simulink model "VVA_pressure_dynamic_basefreq"  (R2023b)
settings: Solver=FixedStepAuto  StartTime=0.0  StopTime=0.6  MaxStep=1e-3  RelTol=1e-3
values from neighbouring files (symbols this model uses):
  x = [2*10^5	3*10^5	4*10^5	5*10^5	6*10^5	7*10^5	8*10^5]    [Q.m]    (also in new_run_compare_export_jieyue.m = ts.Data(:); new_run_compare_sin_export.m = ts.Data(:); objfun_ga.m = double(x(:)); run_compare_jieyue.m = ts.Data(:))
  y = [0 ... (first row only)    [Q.m]    (also in new_run_compare_export_jieyue.m = interp1(t0u, x0u, t(:), method, 'extrap'); new_run_compare_sin_export.m = interp1(t0u, x0u, t(:), method, 'extrap'); objfun_ga.m = y(ia); run_compare_jieyue.m = interp1(t0u, x0u, t(:), method, 'extrap'))
  z = [0.893557423	1.334431826	1.76701406	2.210901891	2.65062	3.098039216	3.535707573 ... (first row only)    [Q.m]
undefined symbols (not defined in the file or in its folder): freq_mode
libraries: fuzblock x2, simulink x2
settings Model: Creator=Administrator  LastModifiedBy=47371
settings SolverCC: MaxConsecutiveMinStep=2  ZeroCrossAlgorithm=Adaptive  AlgebraicLoopSolver=TrustRegion
settings DebuggingCC: MaskedZcDiagnostic=none  IgnoredZcDiagnostic=none  ArithmeticOperatorsInVariantConditions=warning
settings SFSimCC: CustomCodeUndefinedFunction=UseInterfaceOnly

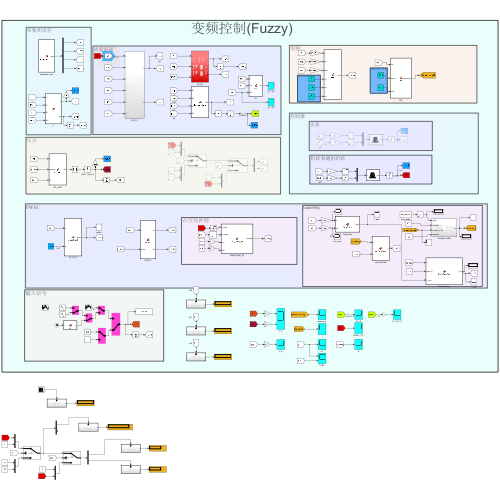
[thumbnail: Simulink's stored preview of the top-level diagram]
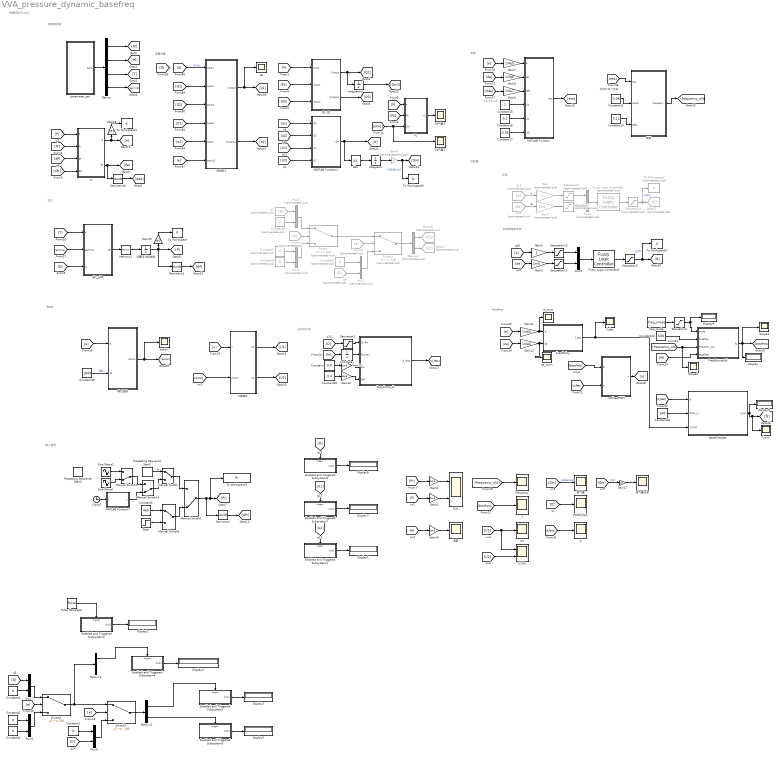
== system VVA_pressure_dynamic_basefreq ==
  note: 输入信号
  note: 占空比补偿
  note: 正弦
  note: 阶跃和随机阶跃
  note: 变频控制(Fuzzy)
  note: 变频
  note: basefrep
  note: 控制器
  note: 压力
  note: 参数和误差
  note: 质量流量
  note: PWM
  note: 变频的两个参数
  note: w1,w2,w3
  2阀模式 : MATLAB Function  TreatAsAtomicUnit=on  SystemSampleTime=0.001
  Abs : Abs  SaturateOnIntegerOverflow=off
  BaseFreqOpt : MATLAB Function  TreatAsAtomicUnit=on
  Clock5 : Clock
  Constant : Constant  Value=0.8
  Constant1 : Constant  Value=4e5
  Constant10 : Constant  Value=1000
  Constant11 : Constant  Value=0.06
  Constant12 : Constant  Value=500
  Constant13 : Constant  Value=500
  Constant14 : Constant  Value=0.12
  Constant15 : Constant
  Constant16 : Constant  Value=0.2
  Constant17 : Constant  Value=0.05
  Constant{2,4..5,8} (4 alike) : Constant  Value=0
  Constant{3,6..7,9} (4 alike) : Constant  Commented=on  Value=0
  Constant32 : Constant  Value=0.4
  Demux : Demux
  Demux1 : Demux  Commented=on  Outputs=2
  Demux2 : Demux  Outputs=2
  Demux3 : Demux  Outputs=2
  Derivative : Derivative
  Derivative1 : Derivative
  Derivative2 : Derivative
  Display{,1..9} (10 alike) : Display
  DutyComp_D : MATLAB Function  TreatAsAtomicUnit=on
  Enabled and Triggered Subsystem1 : Subsystem  TreatAsAtomicUnit=on
  Enabled and Triggered Subsystem2 : Subsystem  TreatAsAtomicUnit=on
  Enabled and Triggered Subsystem3 : Subsystem  TreatAsAtomicUnit=on
  Enabled and Triggered Subsystem4 : Subsystem  TreatAsAtomicUnit=on
  Enabled and Triggered Subsystem5 : Subsystem  TreatAsAtomicUnit=on
  Enabled and Triggered Subsystem7 : Subsystem  TreatAsAtomicUnit=on
  Enabled and Triggered Subsystem8 : Subsystem  TreatAsAtomicUnit=on
  FreqPolicy : MATLAB Function  TreatAsAtomicUnit=on
  FreqSourceSel : Subsystem
  From14 : From  Commented=on  GotoTag=e
  From32 : From  Commented=on  GotoTag=e
  Fuzzy Logic Controller1 : fuzblock/Fuzzy Logic  Controller  Commented=on  FIS="\"fuzzy_pressure_516.fis\""  OutputSampleNumber=101  DataType=double  FuzzifiedInputs=off  RuleFiringStrengths=off  RuleOutputs=off  AggregatedOutputs=off  SimulateUsing=Interpreted execution  OutOfRangeInputValueMessage=warning  NoRuleFiredMessage=warning  EmptyOutputFuzzySetMessage=warning
  Fuzzy Logic Controller3 : fuzblock/Fuzzy Logic  Controller  FIS="\"fuzzy_pressure_516.fis\""  OutputSampleNumber=101  DataType=double  FuzzifiedInputs=off  RuleFiringStrengths=off  RuleOutputs=off  AggregatedOutputs=off  SimulateUsing=Interpreted execution  OutOfRangeInputValueMessage=warning  NoRuleFiredMessage=warning  EmptyOutputFuzzySetMessage=warning
  Gain : Gain  Commented=on
  Gain1 : Gain  Commented=on  Gain=1e-5
  Gain{2,5..6,10,18..19} (6 alike) : Gain  Gain=1e-5
  Gain11 : Gain  Gain=1/4e5
  Gain12 : Gain  Gain=1/3e6
  Gain15 : Gain  Gain=1e-3
  Gain16 : Gain  Gain=1e-3
  Gain17 : Gain  Gain=1/3
  Gain3 : Gain
  Gain4 : Gain  Commented=through  Gain=1/3
  Gain7 : Gain  Gain=1/4e5
  Gain8 : Gain  Gain=1/3e6
  Gain9 : Gain  Gain=1/5e7
  Goto11 : Goto  Commented=on  GotoTag=d
  Goto16 : Goto  Commented=on  GotoTag=U1
  Goto17 : Goto  Commented=on  GotoTag=U2
  Integrator : Integrator
  Integrator3 : Integrator
  MATLAB Function : MATLAB Function  TreatAsAtomicUnit=on
  MATLAB Function1 : MATLAB Function  TreatAsAtomicUnit=on
  MATLAB Function7 : MATLAB Function  TreatAsAtomicUnit=on
  Manual Switch : ManualSwitch
  Manual Switch1 : ManualSwitch  CurrentSetting=0
  Manual Switch14 : ManualSwitch  CurrentSetting=0
  Manual Switch3 : ManualSwitch  CurrentSetting=0
  Manual Switch6 : ManualSwitch
  Memory2 : Memory  InitialCondition=10
  Mux{1..3,5} (4 alike) : Mux  Commented=on  Inputs=2
  Mux{4,6..7,9} (4 alike) : Mux  Inputs=2
  PWM占空比 : Scope
  Pulse Generator : DiscretePulseGenerator  PulseType=Time based  Period=0.01  PulseWidth=5
  Q1 Q2 : Subsystem
  Repeating Sequence Stair2 : simulink/Sources/Repeating Sequence Stair  OutValues=[1.01325e5 4e5 3e5 6e5 3.5e5 5e5 4.5e5 2e5].'  tsamp=1  OutMin=[]  OutMax=[]  OutDataTypeStr=double  OutputDataTypeScalingMode=double  OutDataType=fixdt(0,8)  ConRadixGroup=Best Precision: Vector-wise  OutScaling=2^-12
  Repeating Sequence Stair3 : simulink/Sources/Repeating Sequence Stair  OutValues=[1.01325e5 3e5 2e5 5e5 4e5 2.5e5 1.01325e5].'  tsamp=1  OutMin=[]  OutMax=[]  OutDataTypeStr=double  OutputDataTypeScalingMode=double  OutDataType=fixdt(0,8)  ConRadixGroup=Best Precision: Vector-wise  OutScaling=2^-12
  Saturation1 : Saturate  UpperLimit=1  LowerLimit=0
  Saturation10 : Saturate  UpperLimit=4  LowerLimit=-4
  Saturation11 : Saturate  UpperLimit=35  LowerLimit=-35
  Saturation2 : Saturate  UpperLimit=3  LowerLimit=1
  Saturation4 : Saturate  Commented=on  UpperLimit=0.98  LowerLimit=0.1
  Saturation6 : Saturate  Commented=on  UpperLimit=4  LowerLimit=-4
  Saturation7 : Saturate  Commented=on  UpperLimit=35  LowerLimit=-35
  Saturation9 : Saturate  UpperLimit=0.98  LowerLimit=0.1
  Scope3 : Scope
  Scope4 : Scope
  Sine Wave1 : Sin  Amplitude=2.98675e5  Bias=4e5  Frequency=2*pi*0.25  SampleTime=0
  Sine Wave2 : Sin  Amplitude=2.98675e5  Bias=4e5  Frequency=2*pi*0.5  SampleTime=0
  Step : Step  Before=6e5  After=3e5  SampleTime=0
  Switch : Switch  Commented=on  Threshold=100  SaturateOnIntegerOverflow=off  InputSameDT=off
  Switch1 : Switch  Commented=on  Threshold=-100  SaturateOnIntegerOverflow=off  InputSameDT=off
  Switch2 : Switch  Threshold=100  SaturateOnIntegerOverflow=off  InputSameDT=off
  Switch3 : Switch  Threshold=-100  SaturateOnIntegerOverflow=off  InputSameDT=off
  To Workspace : ToWorkspace  VariableName=P  SaveFormat=Timeseries  SampleTime=0.003
  To Workspace1 : ToWorkspace  VariableName=e  SaveFormat=Timeseries  SampleTime=0.003
  To Workspace2 : ToWorkspace  Commented=on  VariableName=d  SaveFormat=Timeseries  SampleTime=0.003
  To Workspace3 : ToWorkspace  VariableName=Pr  SaveFormat=Timeseries  SampleTime=-1
  To Workspace5 : ToWorkspace  VariableName=Q  SaveFormat=Timeseries  SampleTime=0.003
  To Workspace7 : ToWorkspace  VariableName=d  SaveFormat=Timeseries  SampleTime=0.003
  U1 : Scope
  "U1U2 " : Scope  NumInputPorts=2
  Unit Delay : UnitDelay  SampleTime=-1  HasFrameUpgradeWarning=on
  VL : MATLAB Function  TreatAsAtomicUnit=on
  action : Scope
  d : Scope
  dPL_dPR : MATLAB Function  TreatAsAtomicUnit=on
  de_norm : Scope
  e : MATLAB Function  TreatAsAtomicUnit=on
  e_norm : Scope
  f : Scope
  f_des : Scope
  f_out : Scope
  freq_mode : Constant  Value=freq_mode  SampleTime=-1
  frequency : Scope
  parameter_set : MATLAB Function  TreatAsAtomicUnit=on
  q13 : From  Commented=on  GotoTag=e
  q15 : From  Commented=on  GotoTag=de
  q6 : Scope
  q7 : From  Commented=on  GotoTag=D
  q8 : From  Commented=on  GotoTag=D
  varFreqPWM : MATLAB Function  TreatAsAtomicUnit=on
  压力 : Scope  NumInputPorts=2
  模式选择 : MATLAB Function  TreatAsAtomicUnit=on  SystemSampleTime=0.001
  耗气量 : Scope
  耗气量2 : Scope
  耗气量3 : Scope
  耗气量正弦 : Scope
  设置压力起始值 : Integrator  InitialCondition=1.01325e5
  误差 : Scope
  阀滞后1 : Subsystem
  频率 : MATLAB Function  TreatAsAtomicUnit=on
  wires:
  parameter_set/1(para) -> Demux/1
  Demux/1 -> [Ps]
  Demux/2 -> [P0]
  Demux/3 -> [T]
  Demux/4 -> [gamma]
  dPL_dPR/1(dP) -> Memory2/1
  设置压力起始值/1 -> Gain19/1, [P], Derivative1/1
  [gamma] -> dPL_dPR/2(gamma)
  [T] -> dPL_dPR/1(T)
  [Q] -> dPL_dPR/3(Q)
  [P] -> e/1(P)
  Memory2/1 -> 设置压力起始值/1
  MATLAB Function1/1(dm) -> Abs/1, [Q]
  [Ps] -> Q1 Q2/2(Input1)
  [P0] -> Q1 Q2/3(Input2)
  [P] -> Q1 Q2/1(Input)
  Q1 Q2/1(Output) -> Integrator3/1, [Q1]
  Q1 Q2/2(Output1) -> [Q2]
  [d] -> 阀滞后1/1(Input1)  "占空比"
  [Q1] -> 阀滞后1/2(Input2)
  阀滞后1/1(Output) -> q6/1, [q1]
  阀滞后1/2(Output1) -> [q2]
  [e] -> 阀滞后1/6(Input10)
  [U1] -> 阀滞后1/4(Input6)
  [U2] -> 阀滞后1/5(Input7)
  [Q2] -> 阀滞后1/3(Input3)
  [q1] -> MATLAB Function1/1(Q1)
  [q2] -> MATLAB Function1/2(Q2)
  [U2] -> MATLAB Function1/4(U2)
  [Pr] -> e/2(Pr)
  [dPr] -> e/4(dPr)
  [dP] -> e/3(dP)
  e/1(e) -> Gain18/1, [e]
  e/2(de) -> Derivative2/1, [de]
  Derivative1/1 -> [dP]
  Demux1/2 -> Goto17/1
  Mux5/1 -> Switch/1
  From14/1 -> Switch/2
  Constant6/1 -> Mux5/2
  Constant3/1 -> Mux2/1
  MATLAB Function/1(eta) -> [eta]
  Constant14/1 -> 频率/3(beta)
  Constant17/1 -> MATLAB Function/6(w3)
  Constant15/1 -> MATLAB Function/4(w1)
  频率/1(frequency) -> [frequency_old]
  [eta] -> 频率/1(eta)
  Constant16/1 -> MATLAB Function/5(w2)
  Constant11/1 -> 频率/2(alpha)
  Derivative2/1 -> [dde]
  Mux3/1 -> Fuzzy Logic Controller1/1
  q13/1 -> Gain/1  "e"
  q15/1 -> Gain1/1  "de"
  Fuzzy Logic Controller1/1 -> Saturation4/1
  Saturation4/1 -> To Workspace2/1, Goto11/1  "占空比"
  q7/1 -> Mux5/1
  q8/1 -> Mux2/2
  Switch1/1 -> Demux1/1
  From32/1 -> Switch1/2
  Constant7/1 -> Mux1/1
  Constant9/1 -> Mux1/2
  Mux1/1 -> Switch/3
  Switch/1 -> Switch1/1
  Mux2/1 -> Switch1/3
  Saturation6/1 -> Mux3/1
  Saturation7/1 -> Mux3/2
  Gain/1 -> Saturation6/1
  Gain1/1 -> Saturation7/1
  [de] -> Gain2/1
  [e] -> Gain3/1
  Saturation11/1 -> Mux9/2
  Saturation10/1 -> Mux9/1
  Fuzzy Logic Controller3/1 -> Saturation9/1
  Mux9/1 -> Fuzzy Logic Controller3/1
  Gain2/1 -> Saturation11/1
  Gain3/1 -> Saturation10/1
  Abs/1 -> Integrator/1
  Integrator/1 -> Gain4/1
  Gain4/1 -> To Workspace5/1, [Qm]  "正弦Gain1/3"
  Constant/1 -> Gain15/1
  Constant32/1 -> Gain16/1
  Gain15/1 -> DutyComp_D/3(ton)
  Gain16/1 -> DutyComp_D/4(toff)
  Integrator3/1 -> [Qm1]
  [P0] -> VL/2(P0)
  [Qm1] -> 耗气量2/1, VL/3(Qm)
  VL/1(VL) -> 耗气量3/1
  [P] -> VL/1(P)
  Demux1/1 -> Goto16/1
  Enabled and Triggered Subsystem3/1(Out1) -> Display3/1
  Demux2/1 -> Enabled and Triggered Subsystem3/Trigger
  Mux6/1 -> Switch3/3
  Switch2/1 -> Demux3/1, Switch3/1
  Mux4/1 -> Switch2/3
  Constant8/1 -> Mux4/2
  Constant5/1 -> Mux4/1
  [e] -> Switch3/2
  Switch3/1 -> Demux2/1
  [D] -> Mux6/2
  [D] -> Mux7/1
  Constant2/1 -> Mux6/1
  Constant4/1 -> Mux7/2
  [e] -> Switch2/2
  Mux7/1 -> Switch2/1
  Demux2/2 -> Enabled and Triggered Subsystem5/Trigger
  Demux3/1 -> Enabled and Triggered Subsystem4/Trigger
  Enabled and Triggered Subsystem4/1(Out1) -> Display4/1
  Enabled and Triggered Subsystem5/1(Out1) -> Display5/1
  [U1] -> MATLAB Function1/3(U1)
  模式选择/1(action) -> action/1, [action]
  2阀模式/1(U1) -> [U1]
  2阀模式/2(U2) -> [U2]
  [e] -> 模式选择/1(e)
  [action] -> 2阀模式/2(action)
  Enabled and Triggered Subsystem7/1(Out1) -> Display7/1
  Enabled and Triggered Subsystem8/1(Out1) -> Display8/1
  [U2] -> Enabled and Triggered Subsystem1/Trigger
  Enabled and Triggered Subsystem1/1(Out1) -> Display1/1
  Constant10/1 -> 模式选择/2(et)  "参数"
  [U1] -> Enabled and Triggered Subsystem7/Trigger
  [D] -> Enabled and Triggered Subsystem8/Trigger
  Gain5/1 -> 压力/1
  [Pr] -> Gain5/1
  [P] -> Gain6/1
  Gain6/1 -> 压力/2
  Gain10/1 -> 误差/1
  [e] -> Gain10/1
  [frequency_old] -> frequency/1
  [Qm] -> 耗气量/1  "正弦Gain1/3"
  Saturation9/1 -> [D], To Workspace7/1  "占空比"
  [U1] -> "U1U2 "/1, U1/1
  [U2] -> "U1U2 "/2
  [D] -> PWM占空比/1
  [Qm] -> Gain17/1  "正弦"
  Gain17/1 -> 耗气量正弦/1
  Gain18/1 -> To Workspace1/1
  Gain19/1 -> To Workspace/1
  Repeating Sequence Stair2/1 -> Manual Switch/1  "8s"
  Manual Switch1/1 -> Derivative/1, To Workspace3/1, [Pr]
  Derivative/1 -> [dPr]
  Manual Switch/1 -> Manual Switch1/1
  Constant1/1 -> Manual Switch6/1
  Manual Switch3/1 -> Manual Switch14/1
  Manual Switch6/1 -> Manual Switch1/2
  MATLAB Function7/1(y) -> Manual Switch14/2
  Step/1 -> Manual Switch6/2
  Sine Wave2/1 -> Manual Switch3/1
  Manual Switch14/1 -> Manual Switch/2
  Clock5/1 -> MATLAB Function7/1(t)
  Sine Wave1/1 -> Manual Switch3/2
  Pulse Generator/1 -> Enabled and Triggered Subsystem2/Trigger
  Enabled and Triggered Subsystem2/1(Out1) -> Display2/1
  BaseFreqOpt/1(f_out) -> f_out/1, [fs], Display9/1
  Saturation1/1 -> DutyComp_D/1(d_raw)
  [frequency_old] -> Scope4/1, FreqSourceSel/3(frequency_old)
  Constant12/1 -> FreqSourceSel/2(fixedfrep)
  freq_mode/1 -> Saturation2/1
  Saturation2/1 -> FreqSourceSel/1(mode), Display6/1
  FreqSourceSel/1(fs) -> Scope3/1, [basefreq], Display/1
  [basefreq] -> varFreqPWM/1(fs)
  Constant13/1 -> BaseFreqOpt/2(fmax_in)
  [e] -> Gain7/1
  Gain7/1 -> MATLAB Function/1(e)
  [de] -> Gain8/1
  Gain8/1 -> MATLAB Function/2(de)
  Gain9/1 -> MATLAB Function/3(dde)
  [dde] -> Gain9/1
  FreqPolicy/1(f_des) -> BaseFreqOpt/3(f_cmd), f_des/1
  DutyComp_D/1(d_feas) -> [d_feas]
  [d_feas] -> varFreqPWM/2(d)
  [d_feas] -> BaseFreqOpt/1(d)
  [fs] -> FreqSourceSel/4(basefreq)
  Unit Delay/1 -> DutyComp_D/2(fs_prev)
  [D] -> Saturation1/1
  varFreqPWM/1(u) -> [u]
  [u] -> 2阀模式/1(u)
  [d_feas] -> d/1
  [basefreq] -> f/1
  [e] -> Gain11/1
  Gain11/1 -> e_norm/1, FreqPolicy/1(e)
  [de] -> Gain12/1
  [fs] -> Unit Delay/1
  Gain12/1 -> FreqPolicy/2(de), de_norm/1

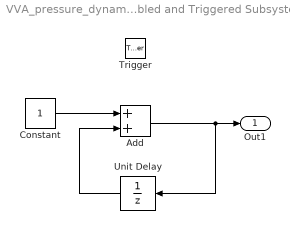
== system VVA_pressure_dynamic_basefreq/Enabled and Triggered Subsystem1 ==
  Trigger : TriggerPort  VariantControl=(inherit)
  Add : Sum
  Constant : Constant
  Unit Delay : UnitDelay  SampleTime=-1  HasFrameUpgradeWarning=on
  Out1 : Outport
  wires:
  Unit Delay/1 -> Add/2
  Add/1 -> Out1/1, Unit Delay/1
  Constant/1 -> Add/1

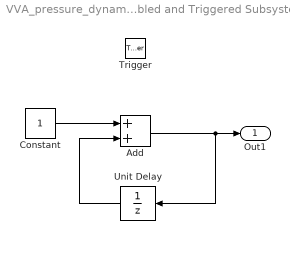
== system VVA_pressure_dynamic_basefreq/Enabled and Triggered Subsystem2 ==
  Trigger : TriggerPort  VariantControl=(inherit)
  Add : Sum
  Constant : Constant
  Unit Delay : UnitDelay  SampleTime=-1  HasFrameUpgradeWarning=on
  Out1 : Outport
  wires:
  Unit Delay/1 -> Add/2
  Add/1 -> Out1/1, Unit Delay/1
  Constant/1 -> Add/1

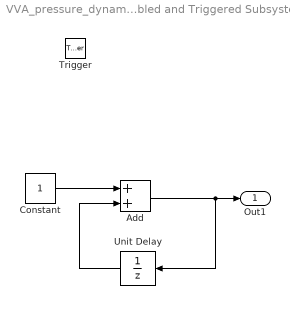
== system VVA_pressure_dynamic_basefreq/Enabled and Triggered Subsystem3 ==
  Trigger : TriggerPort  VariantControl=(inherit)
  Add : Sum
  Constant : Constant
  Unit Delay : UnitDelay  SampleTime=-1  HasFrameUpgradeWarning=on
  Out1 : Outport
  wires:
  Unit Delay/1 -> Add/2
  Add/1 -> Out1/1, Unit Delay/1
  Constant/1 -> Add/1

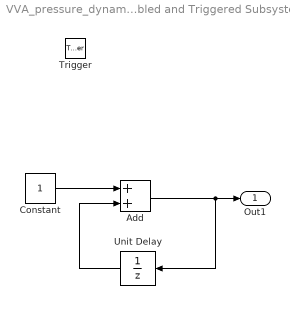
== system VVA_pressure_dynamic_basefreq/Enabled and Triggered Subsystem4 ==
  Trigger : TriggerPort  VariantControl=(inherit)
  Add : Sum
  Constant : Constant
  Unit Delay : UnitDelay  SampleTime=-1  HasFrameUpgradeWarning=on
  Out1 : Outport
  wires:
  Unit Delay/1 -> Add/2
  Add/1 -> Out1/1, Unit Delay/1
  Constant/1 -> Add/1

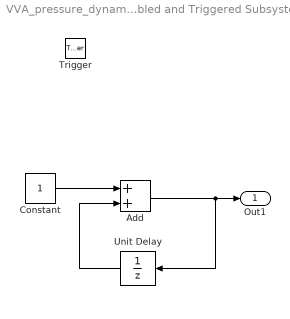
== system VVA_pressure_dynamic_basefreq/Enabled and Triggered Subsystem5 ==
  Trigger : TriggerPort  VariantControl=(inherit)
  Add : Sum
  Constant : Constant
  Unit Delay : UnitDelay  SampleTime=-1  HasFrameUpgradeWarning=on
  Out1 : Outport
  wires:
  Unit Delay/1 -> Add/2
  Add/1 -> Out1/1, Unit Delay/1
  Constant/1 -> Add/1

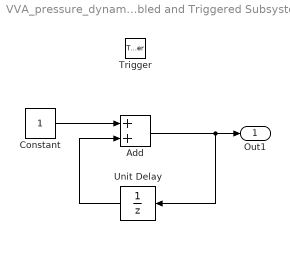
== system VVA_pressure_dynamic_basefreq/Enabled and Triggered Subsystem7 ==
  Trigger : TriggerPort  VariantControl=(inherit)
  Add : Sum
  Constant : Constant
  Unit Delay : UnitDelay  SampleTime=-1  HasFrameUpgradeWarning=on
  Out1 : Outport
  wires:
  Constant/1 -> Add/1
  Add/1 -> Unit Delay/1, Out1/1
  Unit Delay/1 -> Add/2

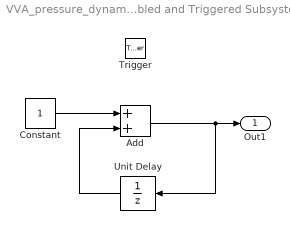
== system VVA_pressure_dynamic_basefreq/Enabled and Triggered Subsystem8 ==
  Trigger : TriggerPort  VariantControl=(inherit)
  Add : Sum
  Constant : Constant
  Unit Delay : UnitDelay  SampleTime=-1  HasFrameUpgradeWarning=on
  Out1 : Outport
  wires:
  Unit Delay/1 -> Add/2
  Add/1 -> Out1/1, Unit Delay/1
  Constant/1 -> Add/1

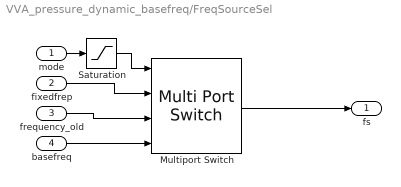
== system VVA_pressure_dynamic_basefreq/FreqSourceSel ==
  mode : Inport
  fixedfrep : Inport  Port=2
  frequency_old : Inport  Port=3
  basefreq : Inport  Port=4
  Multiport Switch : MultiPortSwitch  SaturateOnIntegerOverflow=off  InputSameDT=off
  Saturation : Saturate  UpperLimit=3  LowerLimit=1
  fs : Outport
  wires:
  Multiport Switch/1 -> fs/1
  Saturation/1 -> Multiport Switch/1
  mode/1 -> Saturation/1
  fixedfrep/1 -> Multiport Switch/2
  frequency_old/1 -> Multiport Switch/3
  basefreq/1 -> Multiport Switch/4

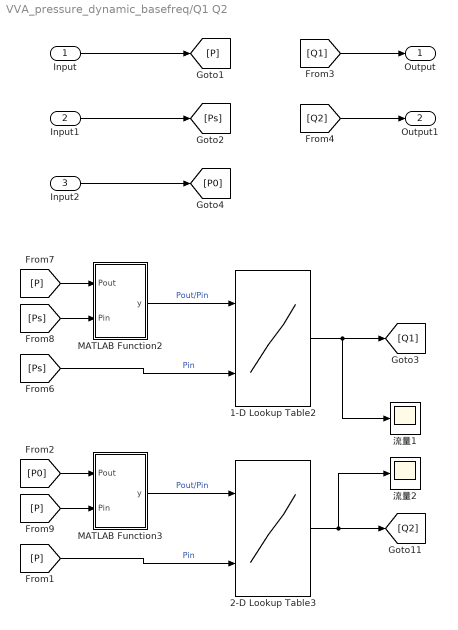
== system VVA_pressure_dynamic_basefreq/Q1 Q2 ==
  Input : Inport
  Input1 : Inport  Port=2
  Input2 : Inport  Port=3
  1-D Lookup Table2 : Lookup_n-D  BreakpointsForDimension1=y  BreakpointsForDimension2=x  Table=z  InterpMethod=Cubic spline  ExtrapMethod=Cubic spline  InternalRulePriority=Speed  RndMeth=Simplest
      settings: InputPortMap=u0,u1
  2-D Lookup Table3 : Lookup_n-D  BreakpointsForDimension1=y  BreakpointsForDimension2=x  Table=z  InterpMethod=Cubic spline  ExtrapMethod=Cubic spline  InternalRulePriority=Speed  RndMeth=Simplest
      settings: InputPortMap=u0,u1
  MATLAB Function2 : MATLAB Function  TreatAsAtomicUnit=on
  MATLAB Function3 : MATLAB Function  TreatAsAtomicUnit=on
  流量1 : Scope
  流量2 : Scope
  Output : Outport
  Output1 : Outport  Port=2
  wires:
  2-D Lookup Table3/1 -> 流量2/1, [Q2]
  [P] -> MATLAB Function2/1(Pout)
  [P0] -> MATLAB Function3/1(Pout)
  MATLAB Function2/1(y) -> 1-D Lookup Table2/1  "Pout/Pin"
  MATLAB Function3/1(y) -> 2-D Lookup Table3/1  "Pout/Pin"
  1-D Lookup Table2/1 -> 流量1/1, [Q1]
  [P] -> MATLAB Function3/2(Pin)
  [Ps] -> MATLAB Function2/2(Pin)
  Input/1 -> [P]
  Input1/1 -> [Ps]
  Input2/1 -> [P0]
  [Q1] -> Output/1
  [Q2] -> Output1/1
  [P] -> 2-D Lookup Table3/2  "Pin"
  [Ps] -> 1-D Lookup Table2/2  "Pin"

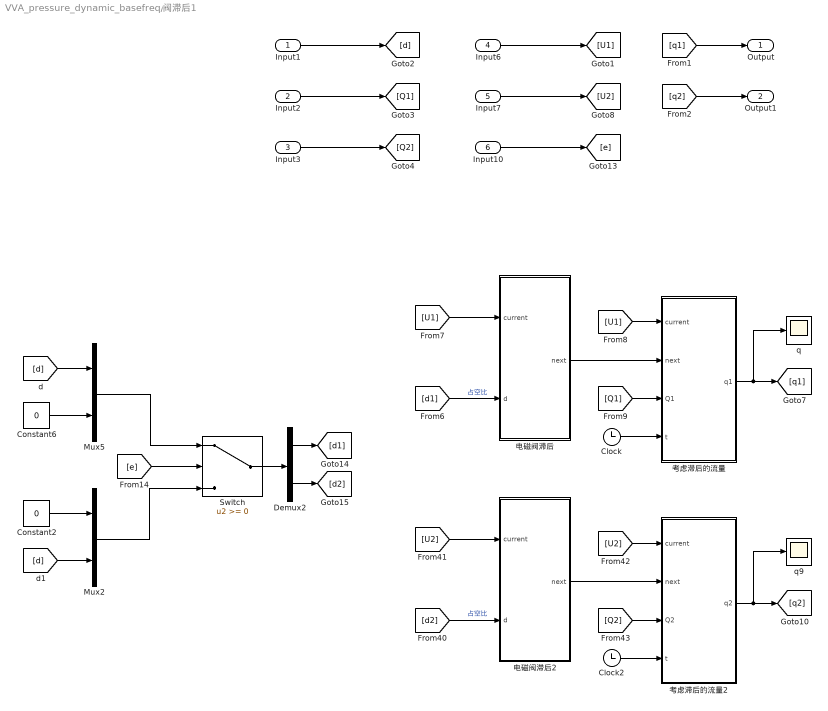
== system VVA_pressure_dynamic_basefreq/阀滞后1 ==
  Input1 : Inport
  Input2 : Inport  Port=2
  Input3 : Inport  Port=3
  Input6 : Inport  Port=4
  Input7 : Inport  Port=5
  Input10 : Inport  Port=6
  " 电磁阀滞后" : MATLAB Function  TreatAsAtomicUnit=on
  " 电磁阀滞后2" : MATLAB Function  TreatAsAtomicUnit=on
  Clock : Clock
  Clock2 : Clock
  Constant2 : Constant  Value=0
  Constant6 : Constant  Value=0
  Demux2 : Demux  Outputs=2
  Mux2 : Mux  Inputs=2
  Mux5 : Mux  Inputs=2
  Switch : Switch  SaturateOnIntegerOverflow=off  InputSameDT=off
  q : Scope
  q9 : Scope
  考虑滞后的流量 : MATLAB Function  TreatAsAtomicUnit=on
  考虑滞后的流量2 : MATLAB Function  TreatAsAtomicUnit=on
  Output : Outport
  Output1 : Outport  Port=2
  wires:
  Clock2/1 -> 考虑滞后的流量2/4(t)
  [U1] -> " 电磁阀滞后"/1(current)
  Clock/1 -> 考虑滞后的流量/4(t)
  [Q1] -> 考虑滞后的流量/3(Q1)
  [d1] -> " 电磁阀滞后"/2(d)  "占空比"
  考虑滞后的流量/1(q1) -> q/1, [q1]
  " 电磁阀滞后"/1(next) -> 考虑滞后的流量/2(next)
  [Q2] -> 考虑滞后的流量2/3(Q2)
  [U1] -> 考虑滞后的流量/1(current)
  考虑滞后的流量2/1(q2) -> [q2], q9/1
  [U2] -> " 电磁阀滞后2"/1(current)
  [d2] -> " 电磁阀滞后2"/2(d)  "占空比"
  " 电磁阀滞后2"/1(next) -> 考虑滞后的流量2/2(next)
  [U2] -> 考虑滞后的流量2/1(current)
  Input1/1 -> [d]
  Input3/1 -> [Q2]
  Input2/1 -> [Q1]
  [q1] -> Output/1
  [q2] -> Output1/1
  Input7/1 -> [U2]
  Input6/1 -> [U1]
  Input10/1 -> [e]
  Mux2/1 -> Switch/3
  Mux5/1 -> Switch/1
  Constant6/1 -> Mux5/2
  [d] -> Mux2/2
  Demux2/1 -> [d1]
  Switch/1 -> Demux2/1
  Constant2/1 -> Mux2/1
  [e] -> Switch/2
  [d] -> Mux5/1
  Demux2/2 -> [d2]

== matlab function VVA_pressure_dynamic_basefreq/BaseFreqOpt ==
  settings: updateMethod=DISCRETE
  data: d input; f_out output; fmax_in input; f_cmd input
function f_out = BaseFreqOpt(d, fmax_in, f_cmd) %#codegen
% PWM基础频率动态优化：物理可行域上限 + 高频预算 + 平滑 + 斜率限制
% 输入:
%   d       : 占空比(0..1)
%   fmax_in : 外部硬上限(Hz)，通常给500
%   f_cmd   : 期望频率(Hz)，来自 FreqPolicy 或 freq门控
% 输出:
%   f_out   : 最终基础频率(Hz)

% ====== 参数区（按你模型需要微调） ======
Ts = 1e-4;          % 必须与 Solver Fixed-step 一致

% 阀运动约束（与你模型一致）
ton  = 0.0008;      % 总开时间(s)
toff = 0.0004;      % 总关时间(s)

kf = 0.94;          % 安全系数(0~1)，越小越保守
f_min = 60;         % 最低频率(Hz)：太低会慢/不稳
f_mid = 160;        % 预算超限时压回的“中频”(Hz)

% 平滑 & 斜率限制
lambda_lp = 0.94;   % 低通滤波(0.90~0.98). 越大越慢越平滑
ramp_up   = 6000;   % 上升最大斜率(Hz/s)
ramp_down = 8000;   % 下降最大斜率(Hz/s)（不要无限快，避免周期突变）

% 高频预算（用来压 nsw：允许短时高频burst，禁止长期高频）
S_max = 18;         % 预算阈值（越小越省开关；过小会影响RMSE）
leak  = 40;         % 预算泄放速度（越大恢复越快）

% ====== 强制标量 & 防御 ======
d      = d(1);
fmax_in = fmax_in(1);
f_cmd  = f_cmd(1);

d = min(max(d,0.0),1.0);
fmax_in = max(fmax_in, 1.0);
f_cmd   = max(f_cmd  , 1.0);

% ====== 物理可行上限：保证 d*T>=ton 且 (1-d)*T>=toff ======
% T = 1/f, 所以 f <= d/ton 且 f <= (1-d)/toff
if (d <= 1e-6) || (d >= 1-1e-6)
    f_upper_phy = f_min; % 极端占空比直接回落到最低可行
else
    f1 = d/max(ton,1e-12);
    f2 = (1-d)/max(toff,1e-12);
    f_upper_phy = kf * min(f1, f2);
end

% 与外部上限合并
f_upper = min(f_upper_phy, fmax_in);
f_lower = min(f_min, f_upper);   % 防止下限>上限

% ====== 目标频率（先限幅） ======
f_tgt = min(max(f_cmd, f_lower), f_upper);

% ====== 高频预算器：抑制长期高频 ======
persistent S f_prev
if isempty(S);      S = 0;      end
if isempty(f_prev); f_prev = f_tgt; end

% 预算累积：高于 f_lower 的部分计入开关“成本”
S = S + max(f_prev - f_lower, 0) * Ts;
% 预算泄放：让系统回到低频后逐渐“恢复额度”
S = max(0, S - leak*Ts);

if S > S_max
    f_tgt = min(f_tgt, f_mid);
end

% ====== 平滑（低通） ======
f_lp = lambda_lp * f_prev + (1 - lambda_lp) * f_tgt;

% ====== 斜率限制（上升慢、下降也有限制避免突变） ======
df = f_lp - f_prev;
df = min(df,  ramp_up  * Ts);
df = max(df, -ramp_down* Ts);
f_out = f_prev + df;

% 最终限幅
f_out = min(max(f_out, f_lower), f_upper);

% 更新记忆
f_prev = f_out;
end

== matlab function VVA_pressure_dynamic_basefreq/MATLAB Function ==
  data: e input; eta output; de input; dde input; w1 input; w2 input; w3 input
function eta = fcn(e,de,dde,w1,w2,w3)   % w1,w2,w3 三个参数 具体大小怎么确定

%w1=1;        %三个参数w1,w2,w3
%w2=0.5;
%w3=1;

eta = w1*e+w2*de+w3*dde;
eta = max(min(eta, 0.5), -0.5);   % 把η夹到[-0.5,0.5]

== matlab function VVA_pressure_dynamic_basefreq/varFreqPWM ==
  settings: updateMethod=DISCRETE
  data: fs input; u output; d input
function u = VarFreqPWM(fs, d) %#codegen
% 可变频PWM（相位累积法）
Ts = 1e-4;  % 与模型 fixed-step 一致

persistent phi
if isempty(phi)
    phi = 0;  % 相位 in [0,1)
end

% 防御
fs = fs(1);
d  = d(1);

fs = max(fs, 1.0);
fs = min(fs, 1e5);
d  = min(max(d,0.0),1.0);

% 相位累积（每步前进 fs*Ts，超过1回绕）
phi = phi + fs*Ts;
phi = phi - floor(phi);

% PWM：phi < d -> 高电平
u = double(phi < d);
end

== matlab function VVA_pressure_dynamic_basefreq/parameter_set ==
  data: para output
function para = parameter_set()  %parameter 变量
global t0_1 t0_2 t0_3 t0_4 flag1 flag2 flag3 flag4;
para = 1:4;  

Ps = 8e5;
P0 = 1.01325e5;
T=  293.15;
gamma =1.4;                



para(1) = Ps;           
para(2) = P0;
para(3) = T;
para(4) = gamma;

== matlab function VVA_pressure_dynamic_basefreq/FreqPolicy ==
  settings: updateMethod=DISCRETE
  data: e input; f_des output; de input
function f_des = FreqPolicy(e, de) %#codegen
% 频率策略：阈值带 + 穿越风险 burst + de低通
% 输入:
%   e  : 归一化误差 e_norm（推荐量级 0~1）
%   de : 归一化误差变化率 de_norm（可能有尖峰，本函数会低通）
% 输出:
%   f_des : 期望频率(Hz)

%% ===== 基本参数（先用这组跑通，再微调） =====
Ts = 1e-4;          % 与模型 fixed-step 一致

% 三档（粗调/中调/精调）
f_low  = 90;        % 大误差：尽量省开关（80~120）
f_mid  = 180;       % 中间误差：中频（150~220）
f_high = 450;       % 小误差精调：较高频（350~500）

% 误差阈值（按 e_norm 量级设置）
E_hi   = 0.45;      % >E_hi 认为还在粗调区（你现在 e_norm≈0.6~0.75，会落在这里）
E_lo   = 0.18;      % <E_lo 进入精调区
E_risk = 0.25;      % 风险判定：接近目标才允许 burst

% de低通（抑制尖峰）
Tf_de  = 0.01;      % 10ms 低通时间常数（可改 0.005~0.03）
a_de   = exp(-Ts/max(Tf_de,1e-12));

% burst 参数
T_burst = 0.03;     % burst 持续时间(s)（20~60ms）
N_burst = max(1, int32(T_burst/Ts));

%% ===== 防御 + 标量化 =====
e  = e(1);
de = de(1);

%% ===== de 低通 =====
persistent de_f
if isempty(de_f)
    de_f = de;
end
de_f = a_de*de_f + (1-a_de)*de;

E = abs(e);

%% ===== 基础频率：阈值带 =====
if E > E_hi
    f_base = f_low;       % 粗调：低频
elseif E > E_lo
    % 在 (E_lo, E_hi) 之间线性插值从 mid -> low
    % E 越大越接近 low，E 越小越接近 mid
    w = (E - E_lo) / max(E_hi - E_lo, 1e-12);   % 0..1
    f_base = f_mid + (f_low - f_mid) * w;
else
    % 精调区：给到较高频，但不直接拉满，留给 burst
    f_base = f_high * 0.75;  % 例如 0.75*450=337.5
end

%% ===== 穿越/超调风险 burst =====
% 风险定义：误差在变小且将要穿越（e*de<0），并且已经接近目标（E<E_risk）
risk = (e*de_f < 0) && (E < E_risk);

persistent burst_cnt
if isempty(burst_cnt)
    burst_cnt = int32(0);
end

if risk
    burst_cnt = N_burst;    % 触发 burst
else
    if burst_cnt > 0
        burst_cnt = burst_cnt - 1;
    end
end

if burst_cnt > 0
    f_des = f_high;         % burst 期间强制高频
else
    f_des = f_base;
end

% 最终防御
f_des = max(f_des, 1.0);
end

== matlab function VVA_pressure_dynamic_basefreq/频率 ==
  settings: updateMethod=DISCRETE
  data: frequency output; eta input; alpha input; beta input
function frequency = fcn(eta, alpha, beta) %#codegen
% 三档变频策略（与Enhancing文献Table I一致）
% 条件：|eta| < alpha -> 高频(500Hz)；alpha<=|eta|<beta -> 中频(300Hz)；|eta|>=beta -> 低频(100Hz)

% --- 强制标量（避免 1-D 向量(1) 传染）---
eta   = eta(1);
alpha = alpha(1);
beta  = beta(1);

A = abs(eta);

% --- 带滞回的档位选择（避免频繁抖动）---
hys = 0;  % 可根据eta量纲调大，如 20~50

persistent level
if isempty(level)
    level = 1; % 1:高频  2:中频  3:低频
end

switch level
    case 1  % 高频
        if A >= alpha + hys
            level = 2;
        end
    case 2  % 中频
        if A < alpha - hys
            level = 1;
        elseif A >= beta + hys
            level = 3;
        end
    case 3  % 低频
        if A < beta - hys
            level = 2;
        end
end

if level == 1
    f_cmd = 500;
elseif level == 2
    f_cmd = 300;
else
    f_cmd = 100;
end

% 轻度平滑（可选）
persistent f_old
if isempty(f_old)
    f_old = f_cmd;
end
lambda_o = 0.90;
f_old = lambda_o * f_old + (1 - lambda_o) * f_cmd;

frequency = f_old;
end

== matlab function VVA_pressure_dynamic_basefreq/MATLAB Function7 ==
  data: t input; y output
function y = fcn(t)

w=0.5*3.14;
% A=167.475;
A=100000;

% y = A*(sin(2*w*t)+sin(w*t)+sin(4*w*t/7)+sin(w*t/3)+sin(4*w*t/17))+400000;
y = A*(sin(2*w*t)+sin(w*t)+sin(0.5*w*t))+400000;

== matlab function VVA_pressure_dynamic_basefreq/DutyComp_D ==
  settings: updateMethod=DISCRETE
  data: d_feas output; d_raw input; fs_prev input; ton input; toff input
function d_feas = DutyComp_D(d_raw, fs_prev, ton, toff) %#codegen
% 把占空比拉回“在当前频率下可实现”的区间：
% d*T >= ton  且 (1-d)*T >= toff

d_raw  = d_raw(1);
fs_prev = fs_prev(1);
ton    = ton(1);
toff   = toff(1);

d_raw = min(max(d_raw,0.0),1.0);
fs_prev = max(fs_prev, 1.0);

T = 1/fs_prev;

d_min = ton / max(T,1e-12);
d_max = 1 - toff / max(T,1e-12);

% 防止不可行区间
d_min = min(max(d_min,0.0),1.0);
d_max = min(max(d_max,0.0),1.0);

if d_min > d_max
    % 极端情况下取中间值
    d_feas = 0.5;
else
    d_feas = min(max(d_raw, d_min), d_max);
end
end

== matlab function VVA_pressure_dynamic_basefreq/阀滞后1/ 电磁阀滞后 ==
  settings: updateMethod=DISCRETE
  data: current input; next output; d input
function next = getNextPWMLevel(current, d)
    % current: 当前PWM信号电平 (0或1)
    % d: 占空比 (0到1之间的值)
    % next: 下一时刻PWM信号电平 (0或1)
    
    if current == 0
        if rand <= d
            next = 1;
        else
            next = 0;
        end
    else
        if rand <= (1 - d)
            next = 0;
        else
            next = 1;
        end
    end
end

== matlab function VVA_pressure_dynamic_basefreq/阀滞后1/ 电磁阀滞后2 ==
  settings: updateMethod=DISCRETE
  data: current input; next output; d input
function next = getNextPWMLevel(current, d)
    % current: 当前PWM信号电平 (0或1)
    % d: 占空比 (0到1之间的值)
    % next: 下一时刻PWM信号电平 (0或1)
    
    if current == 0
        if rand <= d
            next = 1;
        else
            next = 0;
        end
    else
        if rand <= (1 - d)
            next = 0;
        else
            next = 1;
        end
    end
end

== matlab function VVA_pressure_dynamic_basefreq/阀滞后1/考虑滞后的流量 ==
  data: current input; q1 output; next input; Q1 input; t input
function q1= lag(current,next,Q1,t)
period=0.55e-3; %阀开启或关闭时间

mode = 0;
flag1 = 1;

if (current == 0 && next == 0) || (current == 1 && next == 1)
    mode = 0;%不变模式
end
if current == 0 && next == 1
    mode =1;%上升模式
end
if current == 1 && next == 0
    mode =2;%下降模式
end

switch(mode)
    case 0
        q1   = Q1;  %不动模式，流量保持不变
    case 1         %从0到1，流量缓慢增加
        if flag1 == 1
            t0_1 = t;
            flag1 = 0;
        end
        t1 = t - t0_1;
        if t1<=period
            q1 = Q1/period*t1;
        else
            q1 = Q1;
            flag1 = 1;
        end
        
    case 2         %从1到0，流量缓慢减小
        if flag1 == 1
            t0_1 = t;
           flag1 = 0;
        end
        t1 = t - t0_1;
        
        if t1<=period
            q1 = Q1/period*(period - t1);
        else
            q1 = Q1;
            flag1 = 1;
        end
    otherwise
        q1 = Q1;
end

== matlab function VVA_pressure_dynamic_basefreq/阀滞后1/考虑滞后的流量2 ==
  data: current input; q2 output; next input; Q2 input; t input
function q2= lag(current,next,Q2,t)
period=0.55e-3; %阀开启或关闭时间

mode = 0;
flag2 = 1;

if (current == 0 && next == 0) || (current == 1 && next == 1)
    mode = 0;%不变模式
end
if current == 0 && next == 1
    mode =1;%上升模式
end
if current == 1 && next == 0
    mode =2;%下降模式
end

switch(mode)
    case 0
        q2   = Q2;  %不动模式，流量保持不变
    case 1         %从0到1，流量缓慢增加
        if flag2 == 1
            t0_2 = t;
            flag2 = 0;
        end
        t1 = t - t0_2;
        if t1<=period
            q2 = Q2/period*t1;
        else
            q2 = Q2;
            flag2 = 1;
        end
        
    case 2         %从1到0，流量缓慢减小
        if flag2 == 1
            t0_2 = t;
           flag2 = 0;
        end
        t1 = t - t0_2;
        
        if t1<=period
            q2 = Q2/period*(period - t1);
        else
            q2 = Q2;
            flag2 = 1;
        end
    otherwise
        q2 = Q2;
end

== matlab function VVA_pressure_dynamic_basefreq/Q1 Q2/MATLAB Function3 ==
  data: Pout input; y output; Pin input
function y = fcn(Pout,Pin)

y=Pout/Pin;

== matlab function VVA_pressure_dynamic_basefreq/VL ==
  data: P input; VL output; P0 input; Qm input
function VL= fcn(P,P0,Qm)


rou = 1.293*(P/P0); %密度，不考虑温度变化

VL=Qm*1000/rou ;

== matlab function VVA_pressure_dynamic_basefreq/e ==
  data: P input; e output; Pr input; dP input; dPr input; de output
function [e,de]= fcn(P,Pr,dP,dPr)

e = Pr-P;
de=dPr-dP;

== matlab function VVA_pressure_dynamic_basefreq/Q1 Q2/MATLAB Function2 ==
  data: Pout input; y output; Pin input
function y = fcn(Pout,Pin)

y=Pout/Pin;

== matlab function VVA_pressure_dynamic_basefreq/MATLAB Function1 ==
  data: dm output; Q1 input; Q2 input; U1 input; U2 input
function dm = flow_calculate(Q1,Q2,U1,U2)

 dm =U1*Q1 -U2*Q2;

== matlab function VVA_pressure_dynamic_basefreq/2阀模式 ==
  data: U1 output; U2 output; u input; action input
function [U1,U2] =ontrol(u,action)

switch (action)
    
    case 1       
        U1 = u;   %充气
        U2 = 0;

    case 2
        U1 = 0;   %不动
        U2 = 0;

    case 3    
        U1 = 0;   %放气
        U2 = u;
       
    otherwise
        U1 = 0;
        U2 = 0;    
end

== matlab function VVA_pressure_dynamic_basefreq/dPL_dPR ==
  data: dP output size=1; T input; gamma input; Q input
function dP  = dP_fun(T,gamma,Q)

R=0.287;
V=1.57e-4;

dP = gamma*R*T*Q/V;

== matlab function VVA_pressure_dynamic_basefreq/模式选择 ==
  data: e input; action output; et input
function action= control_test(e,et)
        

if e>et    
    action = 1;      %充气  
else        
       
    if e>=-et && e<=et
         action = 2;    %不动
    else
         if e<-et
               action = 3;   %放气
         else
          action=2;   
        end
    end
end
